simulink model "HW1_3"  (R2022b)
settings: Solver=VariableStepAuto  StartTime=0.0  StopTime=10  FixedStep=0.0001  MaxStep=0.001  RelTol=1e-3
values from neighbouring files (symbols this model uses):
  a_sin = [pi/2; pi/2; 0.2; pi/2]    [HW_par.m]
  Kd = 1000*eye(4)    [HW_par.m]
  Kp = 1000*eye(4)    [HW_par.m]
  omega_sin = 10*[1; 1; 1; 1]    [HW_par.m]
  q_0 = [pi/2;pi/4;0;0]    [HW_par.m]
  q_dot_0 = [0;0;0;0]    [HW_par.m]
undefined symbols (not defined in the file or in its folder): a_filt, b_filt
settings Model: Creator=Alberto  LastModifiedBy=emanuelevitetta
settings SolverCC: MaxConsecutiveMinStep=100000  AlgebraicLoopSolver=TrustRegion
settings DebuggingCC: UnconnectedInputMsg=warning  UnconnectedOutputMsg=warning  UnconnectedLineMsg=warning  SFMachineParentedDataDiag=warning
settings ModelReferenceCC: EnableRefExpFcnMdlSchedulingChecks=on
settings RTWCC: DLArmComputeVersion=19.05

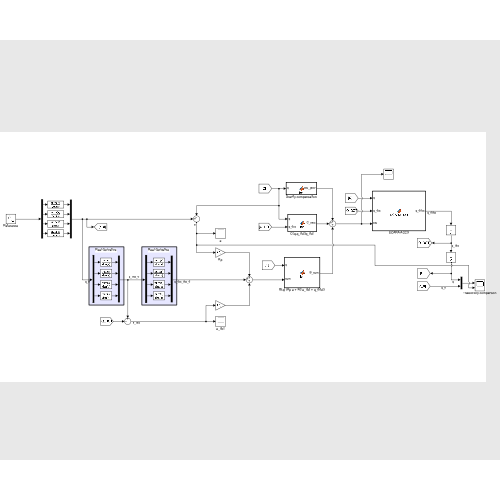
[thumbnail: Simulink's stored preview of the top-level diagram]
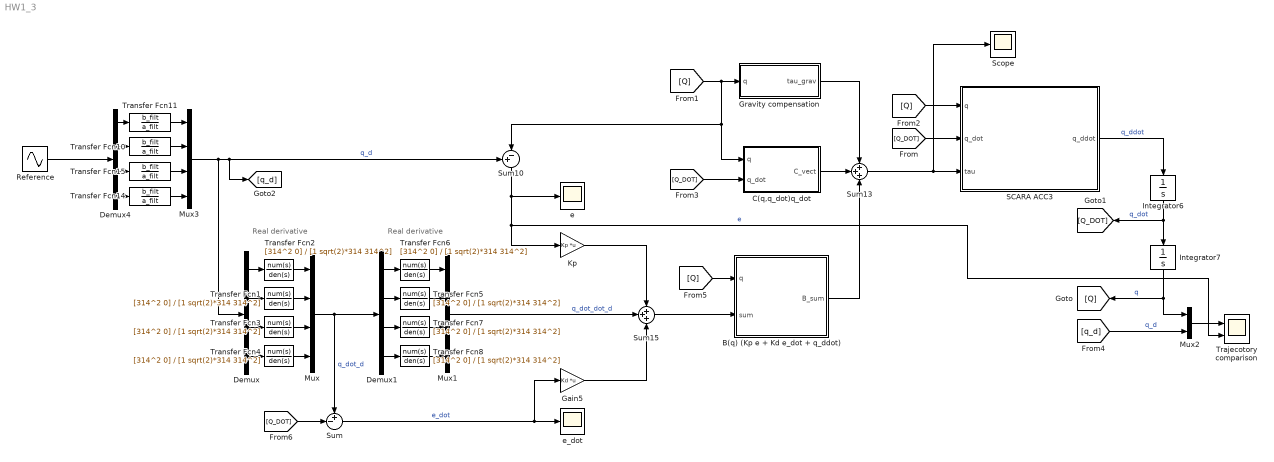
== system HW1_3 ==
  note: Real derivative
  note: Real derivative
  B(q) (Kp e + Kd e_dot + q_ddot) : MATLAB Function  TreatAsAtomicUnit=on
  C(q,q_dot)q_dot : MATLAB Function  TreatAsAtomicUnit=on
  Demux : Demux
  Demux1 : Demux
  Demux4 : Demux
  Gain5 : Gain  Gain=Kd  Multiplication=Matrix(K*u)
  Gravity compensation : MATLAB Function  TreatAsAtomicUnit=on
  Integrator6 : Integrator  InitialCondition=q_dot_0
  Integrator7 : Integrator  InitialCondition=q_0
  Kp : Gain  Gain=Kp  Multiplication=Matrix(K*u)
  Mux : Mux
  Mux1 : Mux
  Mux2 : Mux  Inputs=2
  Mux3 : Mux
  Reference : Sin  Amplitude=a_sin  Frequency=omega_sin  SampleTime=0.001
  SCARA ACC3 : MATLAB Function  TreatAsAtomicUnit=on
  Scope : Scope
  Sum : Sum  Inputs=+-|
  Sum10 : Sum  Inputs=+-|
  Sum13 : Sum  Inputs=+++
  Sum15 : Sum  Inputs=+++
  Trajecotory comparison : Scope  NumInputPorts=2
  Transfer Fcn{1..8} (8 alike) : TransferFcn  Numerator=[314^2 0]  Denominator=[1 sqrt(2)*314 314^2]
  Transfer Fcn{10..11,14..15} (4 alike) : TransferFcn  Numerator=b_filt  Denominator=a_filt
  e : Scope
  e_dot : Scope
  wires:
  Sum10/1 -> e/1, Trajecotory comparison/2, Kp/1  "e"
  Demux4/3 -> Transfer Fcn15/1
  Integrator6/1 -> Integrator7/1, [Q_DOT]  "q_dot"
  Transfer Fcn11/1 -> Mux3/1
  Transfer Fcn10/1 -> Mux3/2
  Transfer Fcn15/1 -> Mux3/3
  Demux4/1 -> Transfer Fcn11/1
  Demux4/2 -> Transfer Fcn10/1
  Sum/1 -> Gain5/1, e_dot/1  "e_dot"
  Sum15/1 -> B(q) (Kp e + Kd e_dot + q_ddot)/2(sum)
  Transfer Fcn14/1 -> Mux3/4
  B(q) (Kp e + Kd e_dot + q_ddot)/1(B_sum) -> Sum13/3
  Gravity compensation/1(tau_grav) -> Sum13/1
  Sum13/1 -> Scope/1, SCARA ACC3/3(tau)
  Mux1/1 -> Sum15/2  "q_dot_dot_d"
  Demux4/4 -> Transfer Fcn14/1
  C(q,q_dot)q_dot/1(C_vect) -> Sum13/2
  SCARA ACC3/1(q_ddot) -> Integrator6/1  "q_ddot"
  [Q] -> Sum10/2, C(q,q_dot)q_dot/1(q), Gravity compensation/1(q)
  [Q_DOT] -> SCARA ACC3/2(q_dot)
  [Q] -> SCARA ACC3/1(q)
  [Q_DOT] -> C(q,q_dot)q_dot/2(q_dot)
  Demux/2 -> Transfer Fcn1/1
  Transfer Fcn1/1 -> Mux/2
  Demux/4 -> Transfer Fcn4/1
  Demux/1 -> Transfer Fcn2/1
  Mux3/1 -> Demux/1, [q_d], Sum10/1  "q_d"
  Transfer Fcn2/1 -> Mux/1
  Transfer Fcn4/1 -> Mux/4
  Transfer Fcn3/1 -> Mux/3
  Demux/3 -> Transfer Fcn3/1
  Mux/1 -> Demux1/1, Sum/1  "q_dot_d"
  Reference/1 -> Demux4/1
  [q_d] -> Mux2/2  "q_d"
  Integrator7/1 -> Mux2/1, [Q]  "q"
  [Q] -> B(q) (Kp e + Kd e_dot + q_ddot)/1(q)
  Kp/1 -> Sum15/1
  Transfer Fcn6/1 -> Mux1/1
  Transfer Fcn7/1 -> Mux1/3
  Demux1/3 -> Transfer Fcn7/1
  Demux1/4 -> Transfer Fcn8/1
  Transfer Fcn8/1 -> Mux1/4
  Transfer Fcn5/1 -> Mux1/2
  Demux1/1 -> Transfer Fcn6/1
  Demux1/2 -> Transfer Fcn5/1
  Gain5/1 -> Sum15/3
  [Q_DOT] -> Sum/2
  Mux2/1 -> Trajecotory comparison/1

== matlab function HW1_3/B(q) (Kp e + Kd e_dot + q_ddot) ==
  data: q input; B_sum output; sum input
function B_sum = fcn(q, sum)%#codegen
coder.extrinsic('f_B_mex'); 
B = eye(4);
B = full(f_B_mex('f_B',q));
B_sum = B * sum;

== matlab function HW1_3/C(q,q_dot)q_dot ==
  data: q input; q_dot input; C_vect output
function C_vect = fcn(q, q_dot)%#codegen
coder.extrinsic('f_C_vect_mex'); 
C_vect = zeros(4,1);
C_vect = reshape(full(f_C_vect_mex('f_C_vect', q, q_dot)),4 ,1);

== matlab function HW1_3/SCARA ACC3 ==
  data: q input; q_ddot output; q_dot input; tau input
function q_ddot = SCARA_acc(q, q_dot, tau)%#codegen
coder.extrinsic('f_B_mex'); 
coder.extrinsic('f_C_vect_mex'); 
coder.extrinsic('f_g_vect_mex');
B = eye(4);
C_vect = zeros(4,1);
F_g = zeros(4,1);
tau = reshape(tau,4,1);
q_ddot = zeros(4,1);
B = full(f_B_mex('f_B',q));
C_vect = full(f_C_vect_mex('f_C_vect', q, q_dot));
F_g = full(f_g_vect_mex('f_g_vect', q));
q_ddot = (eye(4)/B)*(-C_vect-F_g+tau);

== matlab function HW1_3/Gravity compensation ==
  data: q input; tau_grav output
function tau_grav = fcn(q)%#codegen
coder.extrinsic('f_g_vect_mex');
tau_grav = zeros(4,1);
tau_grav = reshape(full(f_g_vect_mex('f_g_vect', q)),4,1);
